simulink model "tofrom"  (Simulink 6.6)
settings: Solver=FixedStepDiscrete  StartTime=0.0  StopTime=10.0  FixedStep=1  RelTol=1e-3
libraries: tofrom_lib x1
settings Model: Creator=ksmyth  LastModifiedBy=hnine
settings DebuggingCC: MultiTaskCondExecSysMsg=none
settings RTWCC: IncludeERTFirstTime=on

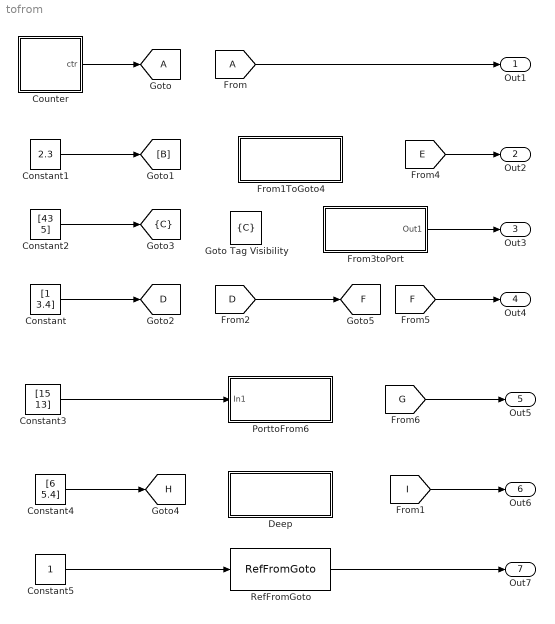
== system tofrom ==
  Constant : Constant  Value=[1 3.4]
  Constant1 : Constant  Value=2.3
  Constant2 : Constant  Value=[43 5]
  Constant3 : Constant  Value=[15 13]
  Constant4 : Constant  Value=[6 5.4]
  Constant5 : Constant
  Counter : Stateflow chart
  Deep : Subsystem
  From1ToGoto4 : Subsystem
  From3toPort : Subsystem
  Goto Tag Visibility : GotoTagVisibility  GotoTag=C
  PorttoFrom6 : Subsystem
  RefFromGoto : tofrom_lib/RefFromGoto  SystemSampleTime=-1
  Out1 : Outport
  Out2 : Outport  Port=2  PortDimensions=[1 1]  DataType=double
  Out3 : Outport  Port=3
  Out4 : Outport  Port=4
  Out5 : Outport  Port=5
  Out6 : Outport  Port=6
  Out7 : Outport  Port=7
  tag scope: A=global, C=scoped, D=global, F=global, H=global
  wires:
  Counter/1(ctr) -> [A]
  [A] -> Out1/1
  Constant1/1 -> [B]
  [E] -> Out2/1
  Constant/1 -> [D]
  [D] -> [F]
  [F] -> Out4/1
  Constant2/1 -> [C]
  From3toPort/1(Out1) -> Out3/1
  Constant3/1 -> PorttoFrom6/1(In1)
  [G] -> Out5/1
  Constant4/1 -> [H]
  [I] -> Out6/1
  Constant5/1 -> RefFromGoto/1
  RefFromGoto/1 -> Out7/1

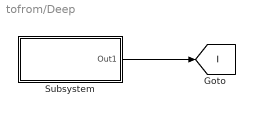
== system tofrom/Deep ==
  Subsystem : Subsystem
  tag scope: I=global
  wires:
  Subsystem/1(Out1) -> [I]

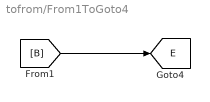
== system tofrom/From1ToGoto4 ==
  tag scope: E=global
  wires:
  [B] -> [E]

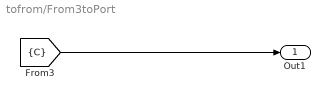
== system tofrom/From3toPort ==
  Out1 : Outport
  wires:
  [C] -> Out1/1

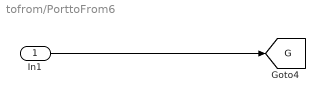
== system tofrom/PorttoFrom6 ==
  In1 : Inport
  tag scope: G=global
  wires:
  In1/1 -> [G]

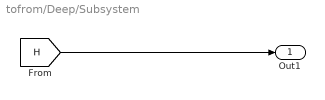
== system tofrom/Deep/Subsystem ==
  Out1 : Outport
  wires:
  [H] -> Out1/1

== stateflow chart Counter ==
  settings: executeAtInitialization=1
  state s1
  (default) -> s1
  s1 -> s1 [order 1] : [ctr < 3] / ctr = ctr+1;
  s1 -> s1 [order 2] : [ctr >= 3] / ctr = 0;
  data: ctr output double =0
